simulink model "main_quad_rev1"  (R2021a)
settings: Solver=FixedStepAuto  StartTime=0.0  StopTime=inf  FixedStep=0.001  RelTol=1e-3
libraries: speedgoatlib_IO691 x5, canmsglib x4, slrealtimeutilitieslib x2
settings Model: SimulationMode=external  NumberOfSteps=2  ExtModeEnableFloating=off  Creator=celwe  LastModifiedBy=johna
settings SolverCC: ConcurrentTasks=on  PositivePriorityOrder=on
settings OptimizationCC: BlockReduction=off  OptimizeBlockIOStorage=off
settings DebuggingCC: TasksWithSamePriorityMsg=none
settings HardwareCC: ProdBitPerLong=64  ProdLongLongMode=on  ProdHWDeviceType=Intel->x86-64 (Linux 64)
settings RTWCC: Description=Simulink Real-Time  SystemTargetFile=slrealtime.tlc  TemplateMakefile=slrealtime_default_tmf  Toolchain=Simulink Real-Time Toolchain  BuildConfiguration=Faster Runs  CodeExecutionProfiling=on  TargetLang=C++

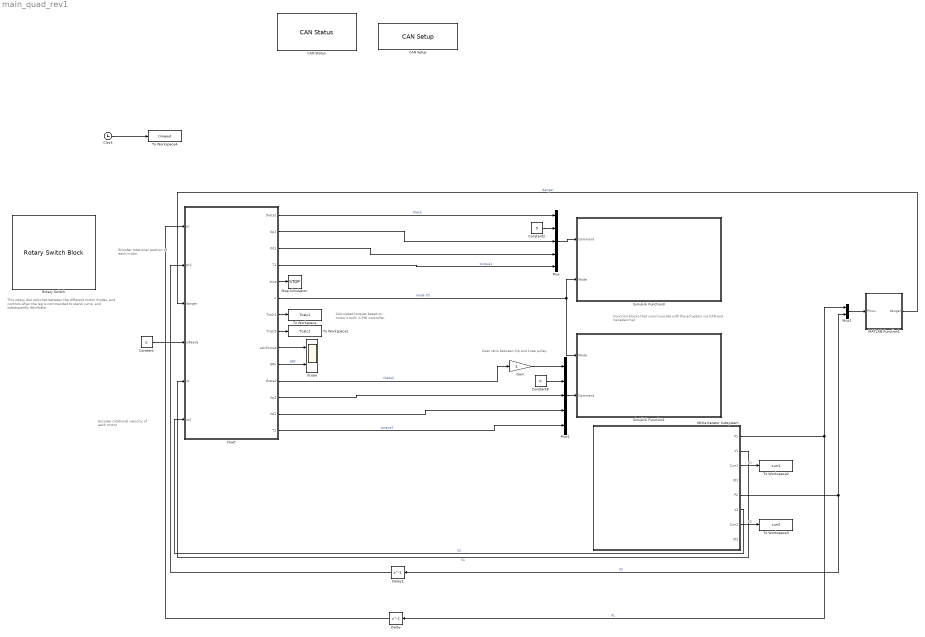
== system main_quad_rev1 ==
  note: Function blocks that communicate with the actuators via CAN
      | and hexadecimal.
  note: Calculated torques based on
      | motor's built in PID controller.
  note: Encoder rotational velocity
      | of each motor
  note: Encoder rotational position
      |  of each motor
  note: Gear ratio between hip and knee pulley
  note: This rotary dial switches between the different motor modes,
      | and controls when the leg is commanded to stand, jump, and
      | subsequently deinitiate.
  "CAN Setup " : speedgoatlib_IO691/CAN Setup   moduletype=IO691  id=1  pciSlot=-1  chn1=CAN (HS)  chn2=CAN (HS)  chn3=Disabled  chn4=Disabled  initStruct=[]  termStruct=[]  ArbitrationbdrChn1=1.0 MBaud  ArbitrationManbdrChn1=[2,8,31,8]  FdbdrChn1=5.0 MBaud  FdManbdrChn1=[2,2,5,2]  ArbitrationbdrChn2=1.0 MBaud  ArbitrationManbdrChn2=[2,8,31,8]  FdbdrChn2=5.0 MBaud  FdManbdrChn2=[2,2,5,2]  ArbitrationbdrChn3=1.0 MBaud  ArbitrationManbdrChn3=[2,8,31,8]  FdbdrChn3=5.0 MBaud  FdManbdrChn3=[2,2,5,2]  ArbitrationbdrChn4=1.0 MBaud  ArbitrationManbdrChn4=[2,8,31,8]  FdbdrChn4=5.0 MBaud  FdManbdrChn4=[2,2,5,2]  moduleInitValues=[691 1 -1 -1]
      settings: SourceProductName=Simulink Real-Time: Speedgoat I/O Blockset
  CAN Status : speedgoatlib_IO691/CAN Status  moduleId=1  sampleTime=-1  channel=1  busRecovery=Off  arrayOutput=off  controllerCpuLoad=off  controllerLiveCount=off  initModeAct=off  avgBusLoad=off  receiving=off  RxQueueEmpty=off  dataOverrunRcv=off  rxBufferLevel=off  txPending=off  dataOverrunTx=off  txBufferLevel=off  errWarnLimit=off  errPassLimit=off  errBusOff=off  busRecoveryCounter=off  busCouplingErr=off  transceiverErr=off  opMode=off  brp=off  timeSegment1=off  timeSegment2=off  synchronisationJumpWidth=off  dataTSEG1=off  dataTSEG2=off  dataSJW=off  moduleType=691  qtyStatBlk=1  ptIdx=0  isFDMod=0
      settings: SourceProductName=Simulink Real-Time: Speedgoat I/O Blockset
  Chart : Stateflow chart  TreatAsAtomicUnit=on
      settings: PortSchema="{\"entries\":[{\"content\":{\"sides\":[{\"content\":{\"connectorIds\":[\"In1\",\"In2\",\"In3\",\"In4\",\"In5\",\"In6\"]},\"type\":\"ConnectorPlacement.EquallySpacedRectSide\",\"uuid\":\"09499f21-f50c-4ce4-914e-8b9942bcc246\"},{\"content\":{\"connectorIds\":[\"Out2\",\"Out7\",\"Out9\",\"Out5\",\"Out1\",\"Out4\",\"Out11\",\"Out12\",\"Out13\",\"Out14\",\"Out3\",\"Out8\",\"Out10\",\"Out6\"],\"side\":\"RIGHT\"},\"type\":\"ConnectorPlacement.EquallySpacedRectSide\",\"uuid\":\"b935e908-ace3-4dfb-ad6d-08dfed6ffdb3\"},{\"content\":{\"connectorIds\":[],\"side\":\"TOP\"},\"type\":\"ConnectorPlacement.EquallySpacedRectSide\",\"uuid\":\"4cd7c5d6-1f1f-4a1f-84b4-9b198395645e\"}]},\"type\":\"ConnectorPlacement.EquallySpacedConnector\",\"uuid\":\"2dc6a8af-05a8-4f21-87ab-6863f156f450\"}],\"packageUris\":[\"http://schema.mathworks.com/mf0/Connector/R2020b\"],\"version\":\"1.0\"}"
  Clock : Clock
  Constant : Constant  Value=0
  Constant2 : Constant  Value=0
  Constant8 : Constant  Value=0
  Delay : Delay  DelayLength=1
  Delay1 : Delay  DelayLength=1
  Gain : Gain
  MATLAB Function1 : MATLAB Function  TreatAsAtomicUnit=on
  Mux : Mux  Inputs=5
  Mux1 : Mux  Inputs=5
  Mux2 : Mux  Inputs=2
  Rotary Switch : RotarySwitchBlock
      settings: Values={{'Zeroing', 'Initiated', 'Stand', 'Jumping', 'deInit', 'Idle'}, [0 1 2 3 4 5]}
  Scope : Scope  NumInputPorts=2
  Simulink Function1 : Subsystem  TreatAsAtomicUnit=on
  Simulink Function3 : Subsystem  TreatAsAtomicUnit=on
  Stop Simulation : Stop
  To Workspace : ToWorkspace  VariableName=Tcalc1  SampleTime=-1
  To Workspace1 : ToWorkspace  VariableName=Tcalc2  SampleTime=-1
  To Workspace2 : ToWorkspace  VariableName=curr1  SampleTime=-1
  To Workspace3 : ToWorkspace  VariableName=curr2  SampleTime=-1
  To Workspace4 : ToWorkspace  VariableName=timeout  SampleTime=-1
  While Iterator Subsystem : Subsystem  TreatAsAtomicUnit=on
  wires:
  Mux/1 -> Simulink Function3/1(Command)
  Chart/7(Kp1) -> Mux/3
  Chart/5(T1) -> Mux/5  "torque1"
  Chart/10(Kd2) -> Mux1/4
  Constant8/1 -> Mux1/2
  Mux1/1 -> Simulink Function1/2(Command)
  Chart/8(Kp2) -> Mux1/3
  Chart/4(c) -> Simulink Function3/2(Mode), Simulink Function1/1(Mode)  "mode (C)"
  Chart/6(T2) -> Mux1/5  "torque2"
  Mux2/1 -> MATLAB Function1/1(Pmux)
  MATLAB Function1/1(danger) -> Chart/3(danger)  "danger"
  Gain/1 -> Mux1/1
  Chart/3(theta2) -> Gain/1  "theta2"
  While Iterator Subsystem/1(P1) -> Delay/1, Mux2/1  "P1"
  While Iterator Subsystem/2(V1) -> Chart/5(vc)  "V1"
  While Iterator Subsystem/3(Curr1) -> To Workspace2/1  "I1"
  While Iterator Subsystem/5(P2) -> Delay1/1, Mux2/2  "P2"
  While Iterator Subsystem/6(V2) -> Chart/6(vc2)  "V2"
  While Iterator Subsystem/7(Curr2) -> To Workspace3/1  "I2"
  Delay/1 -> Chart/1(pc)
  Chart/1(stop) -> Stop Simulation/1
  Delay1/1 -> Chart/2(pc2)
  Constant/1 -> Chart/4(isReady)
  Chart/11(Tcalc1) -> To Workspace/1
  Chart/12(Tcalc2) -> To Workspace1/1
  Clock/1 -> To Workspace4/1
  Chart/13(calcForceX) -> Scope/1
  Chart/14(GRF) -> Scope/2  "GRF"
  Chart/9(Kd1) -> Mux/4
  Constant2/1 -> Mux/2
  Chart/2(theta1) -> Mux/1  "theta"

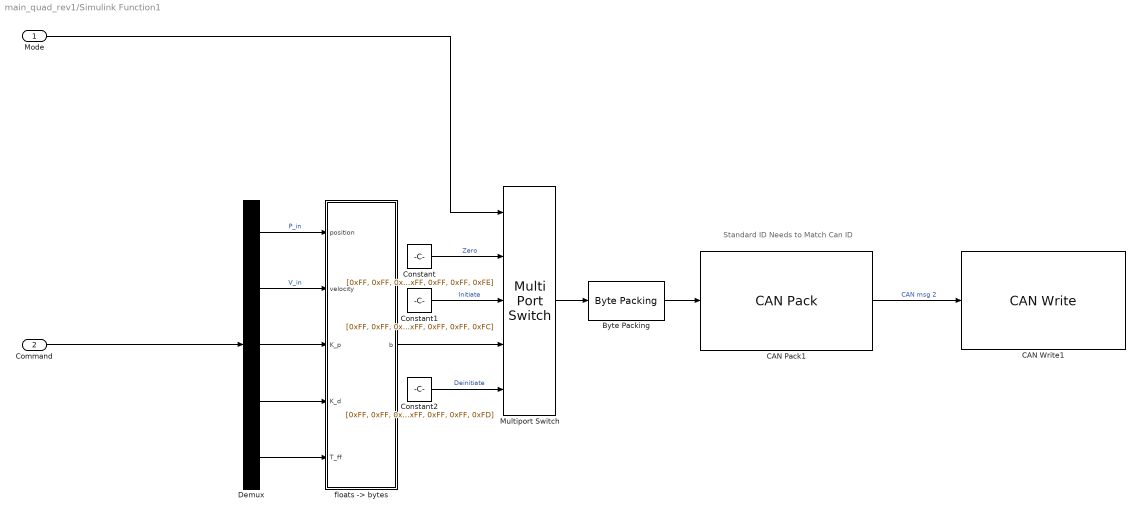
== system main_quad_rev1/Simulink Function1 ==
  note: Standard ID Needs to Match Can ID
  Mode : Inport
  Command : Inport  Port=2
  Byte Packing : slrealtimeutilitieslib/Byte Packing  MaskPackedDataType=uint8  MaskUnpackedDataTypes={['uint8']}  MaskAlignment=1
  CAN Pack1 : canmsglib/CAN Pack  MsgList=(none)  MsgName=CAN Msg  MsgIDType=Standard (11-bit identifier)  MsgIdentifier=8  MsgLength=8  Remote=off  ApplyMinMax=off  BusOutput=off  SignalInfo={ 'b1', '0', '8', 'LE', 'unsigned', 'Standard', '0', '1', '0', '-Inf', 'Inf'; 'b2', '8', '8', 'LE', 'unsigned', 'Standard', '0', '1', '0', '-Inf', 'Inf'; 'b3', '16', '8', 'LE', 'unsigned', 'Standard', '0', '1', '0', '-Inf', 'Inf'; 'b4', '24', '8', 'LE', 'unsigned', 'Standard', '0', '1', '0', '-Inf', 'Inf'; 'b5', '32', '8', 'LE', 'unsigned', 'Standard', '0', '1', '0', '-Inf', 'Inf'; 'b6', '40', '8', 'LE', 'unsigned', 'Standard', '0', '1', '0', '-Inf', 'Inf'; 'b7', '48', '8', 'LE', 'unsigned', 'Standard', '0', '1', '0', '-Inf', 'Inf'; 'b8', '56', '8', 'LE', 'unsigned', 'Standard', '0', '1', '0', '-Inf', 'Inf' }
      settings: SourceProductBaseCode=ME,XP,VN  DataFormat=raw data
  CAN Write1 : speedgoatlib_IO691/CAN Write  id=1  ts=-1  channel=1  messageType=CAN  enableStatusPort=off  canType=CAN (HS)  initValues=[691 1 -1 0 1 1 0]
      settings: SourceProductName=Simulink Real-Time: Speedgoat I/O Blockset
  Constant : Constant  Value=[0xFF, 0xFF, 0xFF, 0xFF, 0xFF, 0xFF, 0xFF, 0xFE]
  Constant1 : Constant  Value=[0xFF, 0xFF, 0xFF, 0xFF, 0xFF, 0xFF, 0xFF, 0xFC]
  Constant2 : Constant  Value=[0xFF, 0xFF, 0xFF, 0xFF, 0xFF, 0xFF, 0xFF, 0xFD]
  Demux : Demux  Outputs=5
  Multiport Switch : MultiPortSwitch  Inputs=4  DiagnosticForDefault=None
  "floats -> bytes" : MATLAB Function  TreatAsAtomicUnit=on
  wires:
  Demux/5 -> "floats -> bytes"/5(T_ff)
  Multiport Switch/1 -> Byte Packing/1
  Demux/4 -> "floats -> bytes"/4(K_d)
  Demux/1 -> "floats -> bytes"/1(position)  "P_in"
  Constant/1 -> Multiport Switch/2  "Zero"
  Demux/2 -> "floats -> bytes"/2(velocity)  "V_in"
  Constant2/1 -> Multiport Switch/5  "Deinitiate"
  CAN Pack1/1 -> CAN Write1/1  "CAN msg 2"
  Byte Packing/1 -> CAN Pack1/1
  Constant1/1 -> Multiport Switch/3  "Initiate"
  "floats -> bytes"/1(b) -> Multiport Switch/4
  Demux/3 -> "floats -> bytes"/3(K_p)
  Mode/1 -> Multiport Switch/1
  Command/1 -> Demux/1

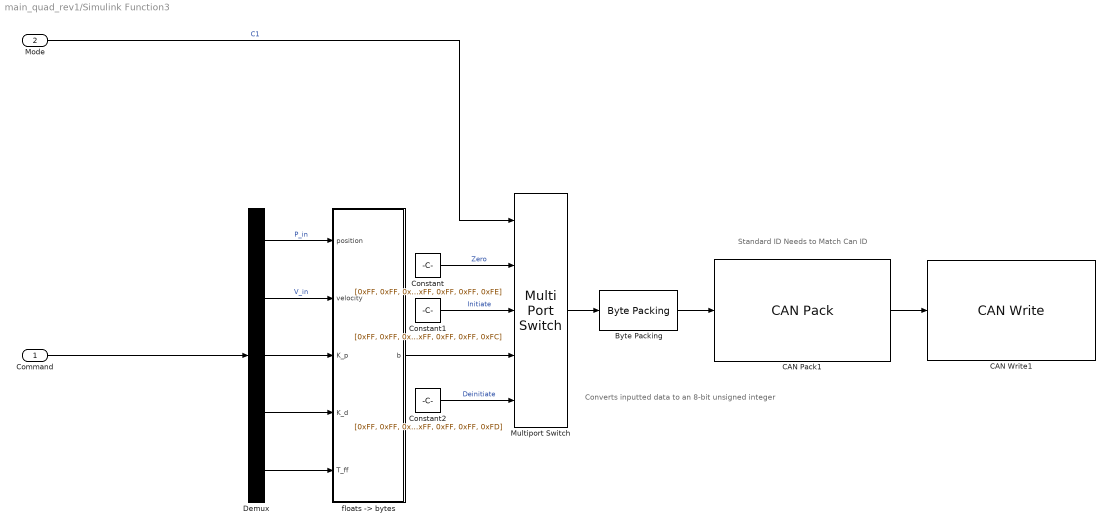
== system main_quad_rev1/Simulink Function3 ==
  note: Standard ID Needs to Match Can ID
  note: Converts inputted data to an 8-bit unsigned integer
  Command : Inport
  Mode : Inport  Port=2
  Byte Packing : slrealtimeutilitieslib/Byte Packing  MaskPackedDataType=uint8  MaskUnpackedDataTypes={['uint8']}  MaskAlignment=1
  CAN Pack1 : canmsglib/CAN Pack  MsgList=(none)  MsgName=CAN Msg  MsgIDType=Standard (11-bit identifier)  MsgIdentifier=7  MsgLength=8  Remote=off  ApplyMinMax=off  BusOutput=off  SignalInfo={ 'b1', '0', '8', 'LE', 'unsigned', 'Standard', '0', '1', '0', '-Inf', 'Inf'; 'b2', '8', '8', 'LE', 'unsigned', 'Standard', '0', '1', '0', '-Inf', 'Inf'; 'b3', '16', '8', 'LE', 'unsigned', 'Standard', '0', '1', '0', '-Inf', 'Inf'; 'b4', '24', '8', 'LE', 'unsigned', 'Standard', '0', '1', '0', '-Inf', 'Inf'; 'b5', '32', '8', 'LE', 'unsigned', 'Standard', '0', '1', '0', '-Inf', 'Inf'; 'b6', '40', '8', 'LE', 'unsigned', 'Standard', '0', '1', '0', '-Inf', 'Inf'; 'b7', '48', '8', 'LE', 'unsigned', 'Standard', '0', '1', '0', '-Inf', 'Inf'; 'b8', '56', '8', 'LE', 'unsigned', 'Standard', '0', '1', '0', '-Inf', 'Inf' }
      settings: SourceProductBaseCode=ME,XP,VN  DataFormat=raw data
  CAN Write1 : speedgoatlib_IO691/CAN Write  id=1  ts=-1  channel=1  messageType=CAN  enableStatusPort=off  canType=CAN (HS)  initValues=[691 1 -1 0 1 1 0]
      settings: SourceProductName=Simulink Real-Time: Speedgoat I/O Blockset
  Constant : Constant  Value=[0xFF, 0xFF, 0xFF, 0xFF, 0xFF, 0xFF, 0xFF, 0xFE]
  Constant1 : Constant  Value=[0xFF, 0xFF, 0xFF, 0xFF, 0xFF, 0xFF, 0xFF, 0xFC]
  Constant2 : Constant  Value=[0xFF, 0xFF, 0xFF, 0xFF, 0xFF, 0xFF, 0xFF, 0xFD]
  Demux : Demux  Outputs=5
  Multiport Switch : MultiPortSwitch  Inputs=4  DiagnosticForDefault=None
  "floats -> bytes" : MATLAB Function  TreatAsAtomicUnit=on
  wires:
  Demux/5 -> "floats -> bytes"/5(T_ff)
  Multiport Switch/1 -> Byte Packing/1
  Demux/4 -> "floats -> bytes"/4(K_d)
  Demux/1 -> "floats -> bytes"/1(position)  "P_in"
  Constant/1 -> Multiport Switch/2  "Zero"
  Demux/2 -> "floats -> bytes"/2(velocity)  "V_in"
  Constant2/1 -> Multiport Switch/5  "Deinitiate"
  CAN Pack1/1 -> CAN Write1/1
  Byte Packing/1 -> CAN Pack1/1
  Constant1/1 -> Multiport Switch/3  "Initiate"
  "floats -> bytes"/1(b) -> Multiport Switch/4
  Demux/3 -> "floats -> bytes"/3(K_p)
  Mode/1 -> Multiport Switch/1  "C1"
  Command/1 -> Demux/1

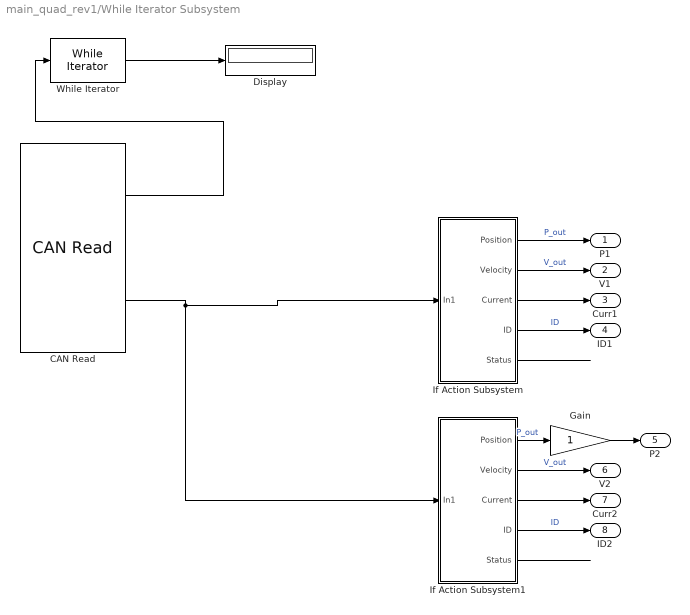
== system main_quad_rev1/While Iterator Subsystem ==
  CAN Read : speedgoatlib_IO691/CAN Read  id=1  ts=-1  channel=1  messageType=CAN  canType=CAN (HS)  initValues=[691 1 -1 0 1 1]
      settings: SourceProductName=Simulink Real-Time: Speedgoat I/O Blockset
  Display : Display
  Gain : Gain
  If Action Subsystem : Subsystem  TreatAsAtomicUnit=on
  If Action Subsystem1 : Subsystem  TreatAsAtomicUnit=on
  While Iterator : WhileIterator  MaxIters=-1  WhileBlockType=do-while  ResetStates=reset  ShowIterationPort=on
  P1 : Outport
  V1 : Outport  Port=2
  Curr1 : Outport  Port=3
  ID1 : Outport  Port=4
  P2 : Outport  Port=5
  V2 : Outport  Port=6
  Curr2 : Outport  Port=7
  ID2 : Outport  Port=8
  wires:
  CAN Read/1 -> While Iterator/1
  CAN Read/2 -> If Action Subsystem1/1(In1), If Action Subsystem/1(In1)
  If Action Subsystem/1(Position) -> P1/1  "P_out"
  If Action Subsystem/2(Velocity) -> V1/1  "V_out"
  If Action Subsystem/3(Current) -> Curr1/1
  If Action Subsystem/4(ID) -> ID1/1  "ID"
  If Action Subsystem/5(Status) -> ?
  If Action Subsystem1/5(Status) -> ?
  If Action Subsystem1/4(ID) -> ID2/1  "ID"
  If Action Subsystem1/3(Current) -> Curr2/1
  If Action Subsystem1/2(Velocity) -> V2/1  "V_out"
  While Iterator/1 -> Display/1
  Gain/1 -> P2/1
  If Action Subsystem1/1(Position) -> Gain/1  "P_out"

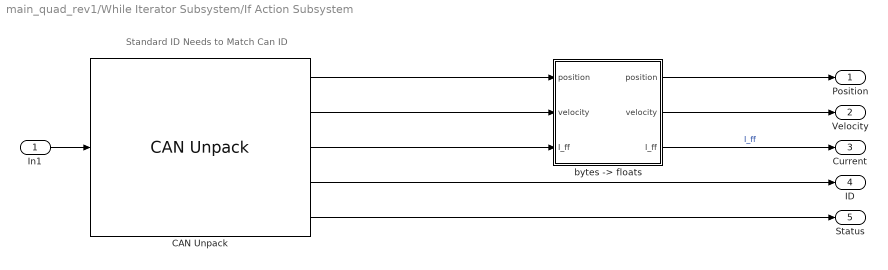
== system main_quad_rev1/While Iterator Subsystem/If Action Subsystem ==
  note: Standard ID Needs to Match Can ID
  In1 : Inport
  CAN Unpack : canmsglib/CAN Unpack  MsgList=(none)  MsgName=CAN Msg  MsgIDType=Standard (11-bit identifier)  MsgIdentifier=7  MsgLength=6  SignalInfo={ 'position', '16', '16', 'BE', 'unsigned', 'Standard', '0', '1', '0', '0', '65535'; 'velocity', '36', '12', 'BE', 'unsigned', 'Standard', '0', '1', '0', '0', '4095'; 'current', '40', '12', 'BE', 'unsigned', 'Standard', '0', '1', '0', '0', '4095'; 'id', '0', '8', 'BE', 'unsigned', 'Standard', '0', '1', '0', '0', '255' }  IDPort=off  TimestampPort=off  ErrorPort=off  RemotePort=off  LengthPort=off  StatusPort=on  ApplyMinMax=off
      settings: SourceProductBaseCode=ME,XP,VN
  "bytes -> floats" : MATLAB Function  TreatAsAtomicUnit=on
  Position : Outport
  Velocity : Outport  Port=2
  Current : Outport  Port=3
  ID : Outport  Port=4
  Status : Outport  Port=5
  wires:
  CAN Unpack/5 -> Status/1
  CAN Unpack/3 -> "bytes -> floats"/3("I_ff ")
  CAN Unpack/4 -> ID/1
  "bytes -> floats"/2(velocity) -> Velocity/1
  "bytes -> floats"/3(I_ff) -> Current/1  "I_ff"
  CAN Unpack/2 -> "bytes -> floats"/2("velocity ")
  In1/1 -> CAN Unpack/1
  CAN Unpack/1 -> "bytes -> floats"/1("position ")
  "bytes -> floats"/1(position) -> Position/1

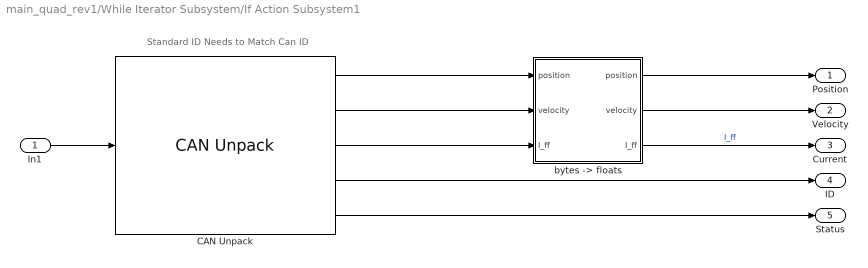
== system main_quad_rev1/While Iterator Subsystem/If Action Subsystem1 ==
  note: Standard ID Needs to Match Can ID
  In1 : Inport
  CAN Unpack : canmsglib/CAN Unpack  MsgList=(none)  MsgName=CAN Msg  MsgIDType=Standard (11-bit identifier)  MsgIdentifier=8  MsgLength=6  SignalInfo={ 'position', '16', '16', 'BE', 'unsigned', 'Standard', '0', '1', '0', '0', '65535'; 'velocity', '36', '12', 'BE', 'unsigned', 'Standard', '0', '1', '0', '0', '4095'; 'current', '40', '12', 'BE', 'unsigned', 'Standard', '0', '1', '0', '0', '4095'; 'id', '0', '8', 'BE', 'unsigned', 'Standard', '0', '1', '0', '0', '255' }  IDPort=off  TimestampPort=off  ErrorPort=off  RemotePort=off  LengthPort=off  StatusPort=on  ApplyMinMax=off
      settings: SourceProductBaseCode=ME,XP,VN
  "bytes -> floats" : MATLAB Function  TreatAsAtomicUnit=on
  Position : Outport
  Velocity : Outport  Port=2
  Current : Outport  Port=3
  ID : Outport  Port=4
  Status : Outport  Port=5
  wires:
  CAN Unpack/5 -> Status/1
  CAN Unpack/1 -> "bytes -> floats"/1("position ")
  CAN Unpack/3 -> "bytes -> floats"/3("I_ff ")
  "bytes -> floats"/1(position) -> Position/1
  CAN Unpack/4 -> ID/1
  "bytes -> floats"/2(velocity) -> Velocity/1
  "bytes -> floats"/3(I_ff) -> Current/1  "I_ff"
  CAN Unpack/2 -> "bytes -> floats"/2("velocity ")
  In1/1 -> CAN Unpack/1

== matlab function main_quad_rev1/While Iterator Subsystem/If Action Subsystem1/bytes -> floats ==
  data: position input; position output; velocity output; I_ff output; velocity input; I_ff input
function [position, velocity, I_ff] = fcn(position, velocity, I_ff)

P_MIN  =-95.5;  % [rad]
P_MAX  = 95.5;  % [rad]
V_MIN  =-45;    % [rad/s]
V_MAX  = 45;    % [rad/s]
I_MIN  =-40;    % []
I_MAX  = 40;    % []

position = position*(P_MAX  - P_MIN)/65535+ P_MIN;
velocity = velocity*(V_MAX  - V_MIN)/4095 + V_MIN;
I_ff     = I_ff*(I_MAX  - I_MIN)/4095 + I_MIN;

== matlab function main_quad_rev1/While Iterator Subsystem/If Action Subsystem/bytes -> floats ==
  data: position input; position output; velocity output; I_ff output; velocity input; I_ff input
function [position, velocity, I_ff] = fcn(position, velocity, I_ff)

P_MIN  =-95.5;  % [rad]
P_MAX  = 95.5;  % [rad]
V_MIN  =-45;    % [rad/s]
V_MAX  = 45;    % [rad/s]
I_MIN  =-40;    % []
I_MAX  = 40;    % []

position = position*(P_MAX  - P_MIN)/65535+ P_MIN;
velocity = velocity*(V_MAX  - V_MIN)/4095 + V_MIN;
I_ff     = I_ff*(I_MAX  - I_MIN)/4095 + I_MIN;

== matlab function main_quad_rev1/Simulink Function1/floats -> bytes ==
  data: position input; b output uint8 size=8; velocity input; K_p input; K_d input; T_ff input
function b = fcn(position, velocity, K_p, K_d, T_ff)

P_MIN  =-95.5;  % [rad]
P_MAX  = 95.5;  % [rad]
V_MIN  =-45;    % [rad/s] 30 to 45
V_MAX  = 45;    % [rad/s]
KP_MIN = 0;     % [Nm/rad]
KP_MAX = 500;   % [Nm/rad]
KD_MIN = 0;     % [Nm*s/rad
KD_MAX = 5;     % [Nm*s/rad
T_MIN  =-18;    % [Nm]
T_MAX  = 18;    % [Nm]

position = floor((max(min(position,P_MAX) ,P_MIN)  - P_MIN )*65535/(P_MAX  - P_MIN));
velocity = floor((max(min(velocity,V_MAX) ,V_MIN)  - V_MIN )*4095 /(V_MAX  - V_MIN));
K_p      = floor((max(min(K_p     ,KP_MAX),KP_MIN) - KP_MIN)*4095 /(KP_MAX - KP_MIN));
K_d      = floor((max(min(K_d     ,V_MAX) ,V_MIN)  - KD_MIN)*4095 /(KD_MAX - KD_MIN));
T_ff     = floor((max(min(T_ff    ,V_MAX) ,V_MIN)  - T_MIN )*4095 /(T_MAX  - T_MIN));

p  = dec2bin(position);
p  = [repmat('0', 1, 16-length(p)),p];
v  = dec2bin(velocity);
v  = [repmat('0', 1, 12-length(v)),v];
kp = dec2bin(K_p);
kp  = [repmat('0', 1, 12-length(kp)),kp];
kd = dec2bin(K_d);
kd  = [repmat('0', 1, 12-length(kd)),kd];
t  = dec2bin(T_ff);
t  = [repmat('0', 1, 12-length(t)),t];

B = repmat('0', 8, 8);

B(1,:) = p(1:8);
B(2,:) = p(9:16);
B(3,:) = v(1:8);
B(4,:) = [v(9:12),kp(1:4)];
B(5,:) = kp(5:12);
B(6,:) = kd(1:8);
B(7,:) = [kd(9:12),t(1:4)];
B(8,:) = t(5:12);

B  = bin2dec(B);

b = uint8(B);

== matlab function main_quad_rev1/Simulink Function3/floats -> bytes ==
  data: position input; b output uint8 size=8; velocity input; K_p input; K_d input; T_ff input
function b = fcn(position, velocity, K_p, K_d, T_ff)

P_MIN  =-95.5;  % [rad]
P_MAX  = 95.5;  % [rad]
V_MIN  =-45;    % [rad/s] 30 to 45
V_MAX  = 45;    % [rad/s]
KP_MIN = 0;     % [Nm/rad]
KP_MAX = 500;   % [Nm/rad]
KD_MIN = 0;     % [Nm*s/rad
KD_MAX = 5;     % [Nm*s/rad
T_MIN  =-18;    % [Nm]
T_MAX  = 18;    % [Nm]

position = floor((max(min(position,P_MAX) ,P_MIN)  - P_MIN )*65535/(P_MAX  - P_MIN));
velocity = floor((max(min(velocity,V_MAX) ,V_MIN)  - V_MIN )*4095 /(V_MAX  - V_MIN));
K_p      = floor((max(min(K_p     ,KP_MAX),KP_MIN) - KP_MIN)*4095 /(KP_MAX - KP_MIN));
K_d      = floor((max(min(K_d     ,V_MAX) ,V_MIN)  - KD_MIN)*4095 /(KD_MAX - KD_MIN));
T_ff     = floor((max(min(T_ff    ,V_MAX) ,V_MIN)  - T_MIN )*4095 /(T_MAX  - T_MIN));

p  = dec2bin(position);
p  = [repmat('0', 1, 16-length(p)),p];
v  = dec2bin(velocity);
v  = [repmat('0', 1, 12-length(v)),v];
kp = dec2bin(K_p);
kp  = [repmat('0', 1, 12-length(kp)),kp];
kd = dec2bin(K_d);
kd  = [repmat('0', 1, 12-length(kd)),kd];
t  = dec2bin(T_ff);
t  = [repmat('0', 1, 12-length(t)),t];

B = repmat('0', 8, 8);

B(1,:) = p(1:8);
B(2,:) = p(9:16);
B(3,:) = v(1:8);
B(4,:) = [v(9:12),kp(1:4)];
B(5,:) = kp(5:12);
B(6,:) = kd(1:8);
B(7,:) = [kd(9:12),t(1:4)];
B(8,:) = t(5:12);

B  = bin2dec(B);

b = uint8(B);

== matlab function main_quad_rev1/MATLAB Function1 ==
  data: Pmux input; danger output
function danger = isDanger(Pmux)
    % Pmux position matrix radians
    %       [p(ID1),p(ID2),p(ID3),p(IDN)]

    
    p1Max = 2; 
    p1Min = -2;
    p2Max = 1.9;
    p2Min = -1.9;
    
    P1 = Pmux(1:2:end);
    P2 = Pmux(2:2:end);
       
    danger = 0;
    if((0<sum([P1>p1Max] + [P1<p1Min] - [P1<=-95.5])) || (0<sum([P2>p2Max] + [P2<p2Min] - [P2<=-95.5])))
        danger = 1;
    end

== stateflow chart main_quad_rev1/Chart ==
  state Start
  state Zero
    entry:
    c = 1;
  state Init
    entry:
    c = 2;
  state Command
    entry:
    c = 3;
    during:
    Tcalc1 = getT(theta1, 0, Kp1, Kd1, T1, pc, vc);
    Tcalc2 = getT(theta2, 0, Kp2, Kd2, T2, pc2, vc2);
    [GRF,calcForceX] = getF(pc, pc2,Tcalc1,Tcalc2);
    state Stand
      entry:
      to = t;
      tstep = 3;
      theta1 = pc;
      po1 = theta1;
      slope1 = (pf - po1)/tstep;
      theta2 = pc2;
      po2 = theta2;
      slope2 = (Th2Th1*pf - po2)/tstep;
      during:
      theta1 = po1 + slope1*(t-to);
      theta2 = po2 + slope2*(t-to);
    state Idle
    state Sit
      entry:
      Kp1 = 25;
      Kp2 = 25;
      Kd1 = 0.1;
      Kd2 = 0.1;
      tstep = 3;
      to = t;
      theta1 = pc;
      po1 = theta1;
      slope1 = (pf - po1)/tstep;
      theta2 = pc2;
      po2 = theta2;
      slope2 = (Th2Th1*pf - po2)/tstep;
      during:
      theta1 = po1 + slope1*(t-to);
      theta2 = po2 + slope2*(t-to);
    (default) -> Stand : {pf = -0.8;}
    Stand -> Idle : [(theta1 >= pf & slope1>0) | (theta1 <= pf & slope1<0)]
        | {theta1 = pf; theta2 = theta1 * Th2Th1;}
    Idle -> Sit : [isReady == 3]{pf = -.8;}
    Sit -> Command : [(theta1 >= pf & slope1>0) | (theta1 <= pf & slope1<0)]
        | {theta1 = pf; theta2 = theta1 * Th2Th1; done = 1;}
  state FinalShutdown
    entry:
    Kp1 = 0;
    Kp2 = 0;
    theta1 = 0;
    theta2 = 0;
    T1 = 0;
    T2 = 0;
  state Deinitiate
    entry:
    c = 4;
  (default) -> Start
  Start -> Init [order 2] : [isReady == 1]
      | {after(3, sec);}
  Start -> Zero [order 1] : [isReady == 0]
  Zero -> Init : [isReady == 1]
      | {after(3,sec);}
  Init -> FinalShutdown [order 2] : [isReady == 4 | danger == 1]
  Init -> Command [order 1] : [isReady == 2]
      | {after(3,sec);}
  Command -> FinalShutdown : [done == 1 | isReady == 4 | danger == 1]
  (junction 36) -> Deinitiate : {stop = 1;}
  Deinitiate -> (junction 36) : after(3,sec)
  FinalShutdown -> Deinitiate
  data: p function_input; v function_input; Kp function_input; Kd function_input; Tff function_input; currP function_input; currV function_input; calcTorque function_output; pos1 function_input; pos2 function_input; Tc1 function_input; Tc2 function_input; calcF function_output; calcFX function_output; stop output =0; theta1 output; theta2 output; c output; done local =0; pc input; pf local; tstep local; to local; pc2 input; T1 output =0; T2 output =0; Kp1 output =25; Kp2 output =25; Kd1 output =.1; Kd2 output =.1; po1 local; po2 local; slope1 local; slope2 local; danger input; isReady input; Tcalc1 output =0; vc input; vc2 input; Tcalc2 output; calcForceX output; GRF output; Th2Th1 local =-1.3
  function calcTorque = getT(p,v,Kp,Kd,Tff,currP,currV):
    | function calcTorque = getT(p,v,Kp,Kd,Tff,currP,currV)
    |     calcTorque = (Kp*(p-currP) + Kd*(v - currV) + Tff);
    | end
  function [calcF,calcFX] = getF(pos1,pos2,Tc1,Tc2):
    | function [calcF,calcFX] = getF(pos1,pos2,Tc1,Tc2)
    |     L1inches = 5.3; %inches
    |     L2inches = 6.36; %inches
    |     L1 = L1inches * 0.0254; %meters
    |     L2 = L2inches * 0.0254; %meters
    | 
    |     J = [(L1 * cos(pos1) + L2 * cos(pos1+pos2)) (L2 * cos(pos1+pos2))
    |          (-L1 * sin(pos1) - L2 * sin(pos1+pos2))  (-L2 * sin(pos1+pos2))];
    |     T = [Tc1;Tc2];
    |     
    |     F = ((J')^-1)*T;
    | 
    |     calcF = F(2);
    |     calcFX = F(1);
    | end
